simulink model "N_scheme_RS"  (R2024b)
settings: Solver=VariableStepAuto  StartTime=0.0  StopTime=10.0  RelTol=1e-3
values from neighbouring files (symbols this model uses):
  b_n = (b_max+b_min)/2    (= 500)    [p20.m]
  Ga = 3    [p20.m]
  Gf = 1/(Gs*Kd)    (= 0.5)    [p20.m]
  Gs = 1    [p20.m]
  K_n = (K_max+K_min)/2    (= 1)    [p20.m]
  Wb = (b_max-b_min)/2    (= 100)    [p20.m]
  Wk = (K_max-K_min)/2    (= 0.6)    [p20.m]
libraries: cstblocks x1
settings Model: Creator=adrian  LastModifiedBy=adrian

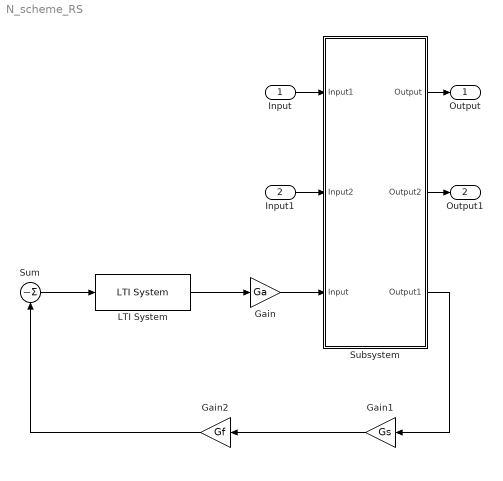
== system N_scheme_RS ==
  Input : Inport
  Input1 : Inport  Port=2
  Gain : Gain  Gain=Ga
  Gain1 : Gain  Gain=Gs
  Gain2 : Gain  Gain=Gf
  LTI System : cstblocks/LTI System  sys=Gc  IC=[]  PadeOrder=0
  Subsystem : Subsystem
  Sum : Sum  Inputs=|-
  Output : Outport
  Output1 : Outport  Port=2
  wires:
  Input/1 -> Subsystem/1(Input1)
  Input1/1 -> Subsystem/2(Input2)
  Gain/1 -> Subsystem/3(Input)
  LTI System/1 -> Gain/1
  Gain1/1 -> Gain2/1
  Subsystem/3(Output1) -> Gain1/1
  Subsystem/1(Output) -> Output/1
  Subsystem/2(Output2) -> Output1/1
  Sum/1 -> LTI System/1
  Gain2/1 -> Sum/1

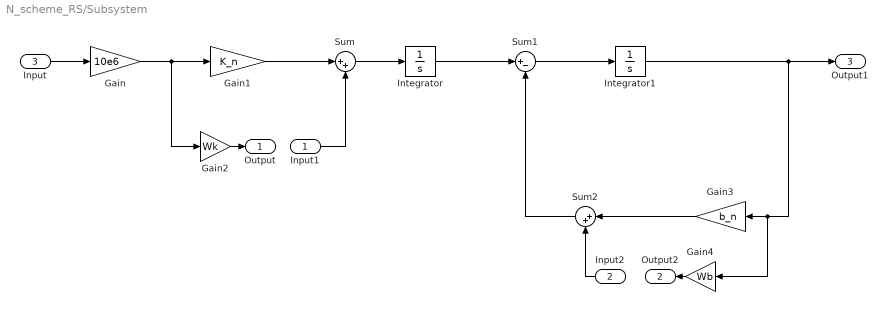
== system N_scheme_RS/Subsystem ==
  Input1 : Inport
  Input2 : Inport  Port=2
  Input : Inport  Port=3
  Gain : Gain  Gain=10e6
  Gain1 : Gain  Gain=K_n
  Gain2 : Gain  Gain=Wk
  Gain3 : Gain  Gain=b_n
  Gain4 : Gain  Gain=Wb
  Integrator : Integrator
  Integrator1 : Integrator
  Sum : Sum  Inputs=|++
  Sum1 : Sum  Inputs=|+-
  Sum2 : Sum  Inputs=|++
  Output : Outport
  Output2 : Outport  Port=2
  Output1 : Outport  Port=3
  wires:
  Gain/1 -> Gain2/1, Gain1/1
  Input/1 -> Gain/1
  Gain1/1 -> Sum/1
  Gain2/1 -> Output/1
  Input1/1 -> Sum/2
  Sum/1 -> Integrator/1
  Integrator/1 -> Sum1/1
  Sum1/1 -> Integrator1/1
  Integrator1/1 -> Gain4/1, Gain3/1, Output1/1
  Gain4/1 -> Output2/1
  Gain3/1 -> Sum2/1
  Input2/1 -> Sum2/2
  Sum2/1 -> Sum1/2
